simulink model "motorCooling"  (R2025b)
settings: Solver=VariableStepAuto  StartTime=0.0  StopTime=80  RelTol=1e-3  AbsTol=1e-3
PreLoadFcn:
  | load fsDCycle.mat
  | vehicleData
undefined symbols (not defined in the file): battery, bevGear, bevMotorSpdRef, cooling, FL, FR, motorDrive, RL, RR, vehicle
libraries: fl_lib x47, nesl_utility x24, sdl_lib x11, SimscapeFluids_lib x3, ee_lib x2, simulink x1, slpidlib x1, autolibshared x1, batteryecm_lib x1, BatteryEstimators x1
(part 1 of 3)
CloseFcn:
  | try,close(h1_ssc_bev_01),end
  | clear h1_ssc_bev_01
  | try,close(h2_ssc_bev_01),end
  | clear h2_ssc_bev_01
  | try,close(h3_ssc_bev_01),end
  | clear h3_ssc_bev_01
  | try,close(h4_ssc_bev_01),end
  | clear h4_ssc_bev_01
  | 
  | 
  | clear simlog_ssc_bev_01
  | clear logsout_ssc_bev_01
Description:
  | Battery Electric Vehicle, Basic Vehicle
settings Model: Creator=smiller  LastModifiedBy=muizz
settings SolverCC: AutoScaleAbsTol=off  MaxConsecutiveMinStep=2  AlgebraicLoopSolver=TrustRegion
settings DataIOCC: MaxDataPoints=10000  ReturnWorkspaceOutputs=off  SignalLoggingName=logsout_motorCooling
settings OptimizationCC: ReuseModelBlockBuffer=off
settings DebuggingCC: UnconnectedInputMsg=warning  UnconnectedOutputMsg=warning  UnconnectedLineMsg=warning  SymbolicDimsDataTypeCodeGenerationDiagnostic=none
settings ModelReferenceCC: EnableRefExpFcnMdlSchedulingChecks=on
settings SFSimCC: CustomCodeUndefinedFunction=UseInterfaceOnly
settings RTWCC: GPUComputeCapability=3.5  DLArmComputeVersion=19.05
settings SimscapeCC: SimscapeLogType=all  SimscapeLogSimulationStatistics=on  SimscapeLogName=simlog_motorCooling  SimscapeLogDataHistory=300000.0

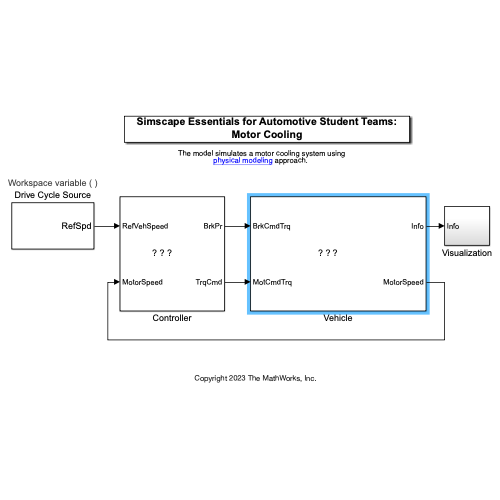
[thumbnail: Simulink's stored preview of the top-level diagram]
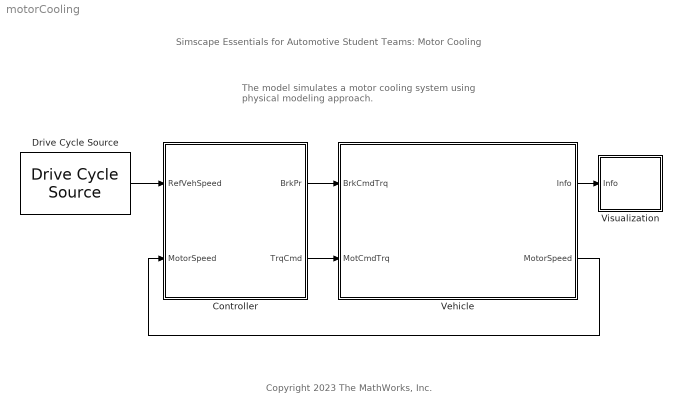
== system motorCooling ==
  note: The model simulates a motor cooling system using physical modeling approach.
  note: Simscape Essentials for Automotive Student Teams: Motor Cooling
  note: Copyright 2023 The MathWorks, Inc.
  Controller : Subsystem
      mask Display: image('Images/brakeThrottle.png'); % Use "Edit Image" on toolstrip to change.
  Drive Cycle Source : autolibshared/Drive Cycle Source  cycleVar=Workspace variable  wsVar=fsdCycle  fileVar=cycleFTP75.mat  tfinal=""  cycleRepeat=on  outAccPort=off  outGearPort=off  gearList=No gear data  t_wot1=5  xdot_woto=0  xdot_wot1=30  t_wot2=20  xdot_wot2=0  t_wotend=30  srcUnit=m/s  outUnit=km/h  srcAccUnit=m/s/s  outAccUnit=m/s^2  dt=0  aMode=1  faultOption=off  velBnd=2  velBndUnit=mph  inUnit=m/s  timeBnd=1  failOption=off  stopSim=off  maxFaultCnt=10  maxFaultTime=2  maxTotFaultTime=15  traceOption=off  dtTrace=1  traceWindow=10  lastDCname=Custom Data Set  lastOutUnit=mph  lastDT=0  lastTB=1  lastSB=2  forceCalcBound=off
  Vehicle : Subsystem
      mask Display: image('Images/vehicle.jpg'); % Use "Edit Image" on toolstrip to change.
  Visualization : Subsystem
  wires:
  Vehicle/2(MotorSpeed) -> Controller/2(MotorSpeed)
  Drive Cycle Source/1 -> Controller/1(RefVehSpeed)
  Vehicle/1(Info) -> Visualization/1(Info)
  Controller/1(BrkPr) -> Vehicle/1(BrkCmdTrq)
  Controller/2(TrqCmd) -> Vehicle/2(MotCmdTrq)

== system motorCooling/Controller ==
  RefVehSpeed : Inport
  MotorSpeed : Inport  Port=2
  Control : Subsystem
      settings: PortSchema="{\"entries\":[{\"content\":{\"sides\":[{\"content\":{\"connectorIds\":[\"Out1\",\"Out2\"]},\"type\":\"ConnectorPlacement.EquallySpacedRectSide\",\"uuid\":\"12b9f2c9-2b28-451b-ad36-7fe4150db485\"},{\"content\":{\"connectorIds\":[\"In1\",\"In2\"],\"side\":\"RIGHT\"},\"type\":\"ConnectorPlacement.EquallySpacedRectSide\",\"uuid\":\"c0fdf9a4-483a-4ddc-b663-6299fcc79327\"},{\"content\":{\"connectorIds\":[],\"side\":\"TOP\"},\"type\":\"ConnectorPlacement.EquallySpacedRectSide\",\"uuid\":\"3f20082e-8487-45e3-9fd7-d6d75741df4d\"}]},\"type\":\"ConnectorPlacement.EquallySpacedConnector\",\"uuid\":\"9361cdd3-74d8-46ee-ae7f-e2dde5d31ed1\"}],\"packageUris\":[\"http://schema.mathworks.com/mf0/Connector/R2020b\"],\"version\":\"1.0\"}"
  Motor Speed Reference : Subsystem
  BrkPr : Outport
  TrqCmd : Outport  Port=2
  tag scope: Ref=global
  wires:
  MotorSpeed/1 -> Control/1(Spd)
  Motor Speed Reference/1(MotorSpdRef) -> Control/2(SpdRef)
  RefVehSpeed/1 -> [Ref], Motor Speed Reference/1(VehSpd)
  Control/1(BrkPr) -> BrkPr/1  "BrkPr"
  Control/2(TrqCmd) -> TrqCmd/1  "MotCmdTrq"

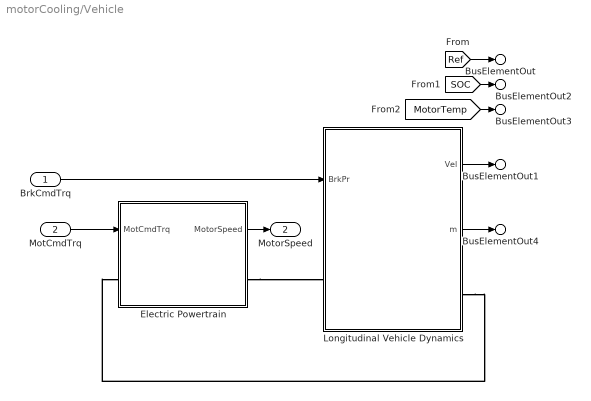
== system motorCooling/Vehicle ==
  BrkCmdTrq : Inport
  MotCmdTrq : Inport  Port=2
  Electric Powertrain : Subsystem
  Longitudinal Vehicle Dynamics : Subsystem
  BusElementOut1 : Outport  PortName=Info  Element=VehSpeed
  BusElementOut : Outport  PortName=Info  Element=RefVehSpeed
  BusElementOut2 : Outport  PortName=Info  Element=SOC
  BusElementOut3 : Outport  PortName=Info  Element=MotorTemp
  BusElementOut4 : Outport  PortName=Info  Element=Vehicle
  MotorSpeed : Outport  Port=2  VectorParamsAs1DForOutWhenUnconnected=off
  wires:
  [Ref] -> BusElementOut/1
  [SOC] -> BusElementOut2/1
  [MotorTemp] -> BusElementOut3/1
  Electric Powertrain/1(MotorSpeed) -> MotorSpeed/1
  BrkCmdTrq/1 -> Longitudinal Vehicle Dynamics/1(BrkPr)
  Longitudinal Vehicle Dynamics/1(Vel) -> BusElementOut1/1
  Longitudinal Vehicle Dynamics/2(m) -> BusElementOut4/1
  MotCmdTrq/1 -> Electric Powertrain/1(MotCmdTrq)
  connections:
  Electric Powertrain/RConn1 -- Longitudinal Vehicle Dynamics/LConn1
  Longitudinal Vehicle Dynamics/RConn1 -- Electric Powertrain/LConn1

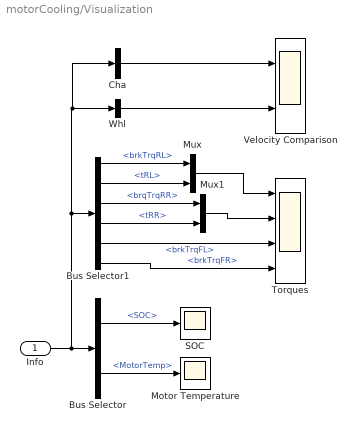
== system motorCooling/Visualization ==
  Info : Inport
  Bus Selector : BusSelector  OutputSignals=SOC,MotorTemp
  Bus Selector1 : BusSelector  OutputSignals=Vehicle.Brakes.RL.brkTrqRL,Vehicle.Chassis.tRL,Vehicle.Brakes.RR.brqTrqRR,Vehicle.Chassis.tRR,Vehicle.Brakes.FL.brkTrqFL,Vehicle.Brakes.FR.brkTrqFR
  Cha : BusSelector  OutputSignals=VehSpeed,RefVehSpeed  OutputAsBus=on
  Motor Temperature : Scope
      settings: ActiveDisplayYMinimum=273.34327  ActiveDisplayYMaximum=321.4106  DataLoggingVariableName=ScopeData3
  Mux : Mux  Inputs=2
  Mux1 : Mux  Inputs=2
  SOC : Scope
      settings: ActiveDisplayYMinimum=0.87315  ActiveDisplayYMaximum=0.90298  DataLoggingVariableName=ScopeData2
  Torques : Scope  NumInputPorts=4
      settings: Title=Rear Left, Brake and Drive Torque  ActiveDisplayYMinimum=-700  ActiveDisplayYMaximum=500
  Velocity Comparison : Scope  NumInputPorts=2
      settings: Title=Vehicle Speed  ActiveDisplayYMinimum=-11.92946  ActiveDisplayYMaximum=107.36516  DataLoggingVariableName=ScopeData2
  Whl : BusSelector  OutputSignals=Vehicle.Brakes.FL.wFL,Vehicle.Brakes.RR.wRR,Vehicle.Brakes.RL.wRL,Vehicle.Brakes.FR.wFR  OutputAsBus=on
  wires:
  Bus Selector/2 -> Motor Temperature/1  "<MotorTemp>"
  Bus Selector/1 -> SOC/1  "<SOC>"
  Whl/1 -> Velocity Comparison/2
  Cha/1 -> Velocity Comparison/1
  Mux1/1 -> Torques/2
  Mux/1 -> Torques/1
  Bus Selector1/4 -> Mux1/2  "<tRR>"
  Bus Selector1/2 -> Mux/2  "<tRL>"
  Bus Selector1/3 -> Mux1/1  "<brqTrqRR>"
  Bus Selector1/1 -> Mux/1  "<brkTrqRL>"
  Bus Selector1/6 -> Torques/4  "<brkTrqFR>"
  Bus Selector1/5 -> Torques/3  "<brkTrqFL>"
  Info/1 -> Cha/1, Whl/1, Bus Selector1/1, Bus Selector/1

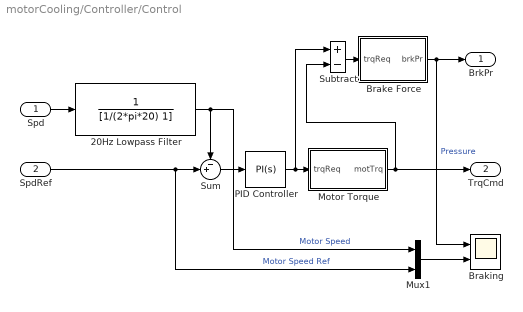
== system motorCooling/Controller/Control ==
  Spd : Inport  Unit=rpm
  SpdRef : Inport  Port=2  Unit=rpm
  20Hz Lowpass Filter : TransferFcn  Denominator=[1/(2*pi*20) 1]
  Brake Force : Subsystem
  Braking : Scope  NumInputPorts=2
      settings: ActiveDisplayYMinimum=-6.26637814618E+6  ActiveDisplayYMaximum=5.639740331562E+7
  Motor Torque : Subsystem
  Mux1 : Mux  Inputs=2
  PID Controller : slpidlib/PID Controller  Controller=PI  Form=Parallel  TimeDomain=Continuous-time  UseExternalTs=off  SampleTime=-1  IntegratorMethod=Forward Euler  FilterMethod=Forward Euler  ControllerParametersSource=internal  P=0.5  I=1e-3  UseKiTs=off  D=0  UseExternalDerivativeSource=off  N=100  UseFilter=on  TunerSelectOption=Transfer Function Based (PID Tuner App)  InitialConditionSource=internal  InitialConditionForIntegrator=0  InitialConditionForFilter=0  DifferentiatorICPrevScaledInput=0  ExternalReset=none  TrackingMode=off  Kt=1  LimitOutput=off  SatLimitsSource=internal  UpperSaturationLimit=inf  LowerSaturationLimit=-inf  LinearizeAsGain=on  AntiWindupMode=none  Kb=1  LimitIntegrator=off  UpperIntegratorSaturationLimit=inf  LowerIntegratorSaturationLimit=-inf  POutMin=[]  POutMax=[]  IOutMin=[]  IOutMax=[]  DOutMin=[]  DOutMax=[]  NOutMin=[]  NOutMax=[]  SumOutMin=[]  SumOutMax=[]  SaturationOutMin=[]  SaturationOutMax=[]  PParamMin=[]  PParamMax=[]  IParamMin=[]  IParamMax=[]  DParamMin=[]  DParamMax=[]  NParamMin=[]  NParamMax=[]  KbParamMin=[]  KbParamMax=[]  KtParamMin=[]  KtParamMax=[]  KbOutMin=[]  KbOutMax=[]  KtOutMin=[]  KtOutMax=[]  IntegratorOutMin=[]  IntegratorOutMax=[]  FilterOutMin=[]  FilterOutMax=[]  SumI1OutMin=[]  SumI1OutMax=[]  SumI2OutMin=[]  SumI2OutMax=[]  SumI3OutMin=[]  SumI3OutMax=[]  SumI4OutMin=[]  SumI4OutMax=[]  SumDOutMin=[]  SumDOutMax=[]  DifferentiatorOutMin=[]  DifferentiatorOutMax=[]  FilterDiffOutCoefMin=[]  FilterDiffOutCoefMax=[]  ReciprocalOutMin=[]  ReciprocalOutMax=[]  SumDenOutMin=[]  SumDenOutMax=[]  SumNumOutMin=[]  SumNumOutMax=[]  DivideOutMin=[]  DivideOutMax=[]  UdiffTsProdOutMin=[]  UdiffTsProdOutMax=[]  NTsProdOutMin=[]  NTsProdOutMax=[]  UintegralTsProdOutMin=[]  UintegralTsProdOutMax=[]  UngainTsProdOutMin=[]  UngainTsProdOutMax=[]  ClampingZeroOutDataTypeStr=Inherit: Inherit via back propagation  ClampingZeroOutMin=[]  ClampingZeroOutMax=[]  FilterDenConstantOutDataTypeStr=Inherit: Inherit via back propagation  FilterDenConstantOutMin=[]  FilterDenConstantOutMax=[]  PCopyOutDataTypeStr=Inherit: Inherit via back propagation  PCopyOutMin=[]  PCopyOutMax=[]  NCopyOutDataTypeStr=Inherit: Inherit via back propagation  NCopyOutMin=[]  NCopyOutMax=[]  IntegratorContinuousStateAttributes=''  IntegratorStateMustResolveToSignalObject=off  IntegratorRTWStateStorageClass=Auto  FilterContinuousStateAttributes=''  FilterStateMustResolveToSignalObject=off  FilterRTWStateStorageClass=Auto  ParallelPVariant=InternalParameters  IdealPVariant=Disabled  IVariant=InternalParameters  DVariant=Disabled  IntegratorVariant=Continuous  SatVariant=Disabled  AWVariant=Passthrough  PCopyVariant=Disabled  TRVariant=Disabled  FdbkBlocksVariant=Forward  IdealPFdbkVariant=Disabled  SatFdbkVariant=Disabled  DerivativeFilterVariant=Disabled  NVariant=Disabled  NCopyVariant=Disabled_SignalSpec  FilterICVariant=Disabled  IntegratorICVariant=InternalICs  ExternalResetVariant=Disabled  TRSumVariant=Passthrough  SumFdbkVariant=Disabled  SumVariant=Sum_PI  TsampFilterVariant=InternalTs  TsampNgainVariant=Passthrough  TsampIntegralVariant=Disabled_SignalSpec  ExternalSaturationOutDataTypeStr=Inherit: Same as second input  DerivativeSourceVariant=Disabled  PreIntVariant=InternalPreInt
  Subtract : Sum  Inputs=+-
  Sum : Sum  Inputs=-+|
  BrkPr : Outport
  TrqCmd : Outport  Port=2  Unit=N*m  VectorParamsAs1DForOutWhenUnconnected=off
  wires:
  20Hz Lowpass Filter/1 -> Sum/1, Mux1/1  "Motor Speed"
  Sum/1 -> PID Controller/1
  Spd/1 -> 20Hz Lowpass Filter/1
  SpdRef/1 -> Mux1/2, Sum/2  "Motor Speed Ref"
  Motor Torque/1(motTrq) -> Subtract/2, TrqCmd/1
  Brake Force/1(brkPr) -> BrkPr/1, Braking/1  "Pressure"
  Subtract/1 -> Brake Force/1(trqReq)
  Mux1/1 -> Braking/2
  PID Controller/1 -> Subtract/1, Motor Torque/1(trqReq)

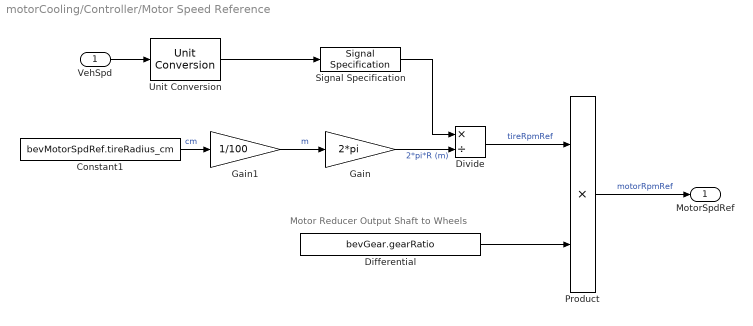
== system motorCooling/Controller/Motor Speed Reference ==
  note: Motor Reducer Output Shaft to Wheels
  VehSpd : Inport  Unit=km/hr
  Constant1 : Constant  Value=bevMotorSpdRef.tireRadius_cm
  Differential : Constant  Value=bevGear.gearRatio
  Divide : Product  Inputs=*/
  Gain : Gain  Gain=2*pi
  Gain1 : Gain  Gain=1/100
  Product : Product
  Signal Specification : SignalSpecification  Unit=m/min
  Unit Conversion : UnitConversion
  MotorSpdRef : Outport  Unit=rpm  VectorParamsAs1DForOutWhenUnconnected=off
  wires:
  VehSpd/1 -> Unit Conversion/1
  Unit Conversion/1 -> Signal Specification/1
  Signal Specification/1 -> Divide/1
  Constant1/1 -> Gain1/1  "cm"
  Gain/1 -> Divide/2  "2*pi*R (m)"
  Divide/1 -> Product/1  "tireRpmRef"
  Product/1 -> MotorSpdRef/1  "motorRpmRef"
  Gain1/1 -> Gain/1  "m"
  Differential/1 -> Product/2

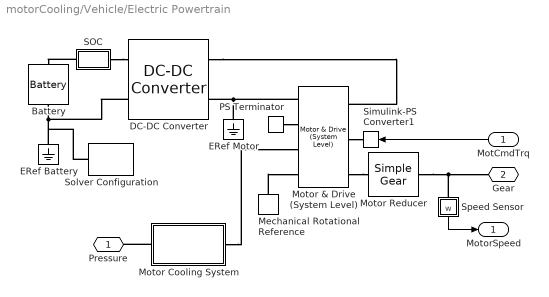
== system motorCooling/Vehicle/Electric Powertrain ==
  MotCmdTrq : Inport
  Battery : batteryecm_lib/Battery  Vnom=battery.voltage_V V  prm_dir=simscape.enum.battery.prm_dir.disabled  R1_dis=2 Ohm  R1_ch=2 Ohm  R1=2e-3 Ohm  prm_AH=simscape.enum.battery.prm_AH.finite  AH=battery.cell_capacity A*hr  V1=battery.voltage_V*11.5/12 V  AH1=10 A*hr  prm_R2=simscape.enum.battery.prm_R2.disabled  R2=2000 Ohm  Tmeas=298.15 K  charge_measurement_port=simscape.enum.battery.enable.no  prm_dyn=simscape.enum.battery.prm_dyn.off  Rp1=0.005 Ohm  tau1=30 s  Rp2=0.005 Ohm  tau2=30 s  Rp3=0.005 Ohm  tau3=30 s  Rp4=0.005 Ohm  tau4=30 s  Rp5=0.005 Ohm  tau5=30 s  prm_fade=simscape.enum.battery.prm_fade.disabled  N_fade=100  AH_fade=45 A*hr  R1_fade=2.02 Ohm  R1_ch_fade=2.02 Ohm  V1_fade=10.35 V  prm_age=simscape.enum.battery.prm_age.disabled  prm_age_OCV=simscape.enum.battery.prm_age_OCV.OCV  OCV_age=0.9  SOC_age=60  Tmeas_age=298.15 K  delta_time_age_vec=[0] d  temperature_age_vec=[273] K  OCV_scaling_age=2.2134e6  OCV_offset_age=1.632e6  temp_exp_age=0.515833569 V  t_exp_age=0.75  Vnom_T2=12 V  R1_T2=2.2 Ohm  R1_T2_dis=2.2 Ohm  R1_T2_ch=2.2 Ohm  V1_T2=11.4 V  R2_T2=2200 Ohm  Rp1_T2=0.005 Ohm  tau1_T2=30 s  Rp2_T2=0.005 Ohm  tau2_T2=30 s  Rp3_T2=0.005 Ohm  tau3_T2=30 s  Rp4_T2=0.005 Ohm  tau4_T2=30 s  Rp5_T2=0.005 Ohm  tau5_T2=30 s  Tmeas2=273.15 K  thermal_port=simscape.enum.thermaleffects.omit  thermal_mass=30000 J/K  i_specify=off  i_priority=None  i=0 A  i_nominal_specify=off  i_nominal_value=1  i_nominal_unit=A  v_specify=off  v_priority=None  v=0 V  v_nominal_specify=off  v_nominal_value=1  v_nominal_unit=V  charge_specify=on  charge_priority=High  charge=battery.cell_capacity*battery.init_soc A*hr  charge_nominal_specify=off  charge_nominal_value=1  charge_nominal_unit=A*hr  num_cycles_specify=off  num_cycles_priority=High  num_cycles=0  num_cycles_nominal_specify=off  num_cycles_nominal_value=1  num_cycles_nominal_unit=1  temperature_specify=off  temperature_priority=High  temperature=298.15 K  temperature_nominal_specify=off  temperature_nominal_value=1  temperature_nominal_unit=K
  DC-DC Converter : ee_lib/Semiconductors & Converters/Converters/DC-DC Converter  Vref_option=ee.enum.converters.voltageref.internal  v_ref=converter.outputVoltage V  P_rated=converter.outputPower W  droop_enabled=true  droop_param=ee.enum.converters.droop.percent  droop=0.1 V/A  droop_percent=converter.droopPercent  Vref_droop=10 V  reversible=ee.enum.converters.directionality.bidirectional  G_diode=1e-8 1/Ohm  P_fixed=1 W  losses_option=ee.enum.converters.lossesOption.proportionalToSquaredCurrent  eff_rated=80  tableOption=ee.enum.converters.lossTableOptionThermal.currentTemp  i_eff_vec=[-2, -1, 1, 2] A  v_eff_vec=[15, 30, 45] V  eff_vec=[66, 76, 80, 74]  eff_2D_table=[66, 66, 66; 76, 76, 76; 80, 80, 80; 74, 74, 74]  model_dynamics=ee.enum.converters.dynamics.no  tau=0.02 s  v_ini=10 V  v1_min=1 V  R1=1000 Ohm  R2=1000 Ohm  fault_condition=ee.enum.faults.faultInputCondition.greaterThan  fault_threshold=0.5  T_eff_vec=[280, 300, 320] K  eff_3D_table=repmat([66; 76; 80; 74], 1, 3, 3)  thermal_mass=100 J/K  initial_temperature=298.15 K
      settings: InternalSimscapePortConfiguration="{\"Bottom\":[],\"Left\":[{\"id\":\"p1\",\"label\":\"1+\",\"type\":\"foundation.electrical.electrical\"},{\"id\":\"n1\",\"label\":\"1-\",\"type\":\"foundation.electrical.electrical\"}],\"Right\":[{\"id\":\"p2\",\"label\":\"2+\",\"type\":\"foundation.electrical.electrical\"},{\"id\":\"n2\",\"label\":\"2-\",\"type\":\"foundation.electrical.electrical\"}],\"Top\":[]}"
  ERef Battery : fl_lib/Electrical/Electrical Elements/Electrical Reference
  ERef Motor : fl_lib/Electrical/Electrical Elements/Electrical Reference
  Mechanical Rotational Reference : fl_lib/Mechanical/Rotational Elements/Mechanical Rotational Reference
  Motor Reducer : sdl_lib/Gears/Simple Gear  ratio=motorDrive.gearRatioCompensation  rotation_direction=3-2*(1)  friction_model=sdl.enum.gear_efficiencies_load.off  T_noload=0.1 N*m  T_nom=5 N*m  efficiency_nom=0.8  efficiency=0.8  temperature_TLU=[280, 300, 320] K  load_TLU=[1, 5, 10] N*m  efficiency_TLU=[.95, .9, .85]  efficiency_TLU2=[.85, .8, .75; .95, .9, .85; .85, .8, .7]  w_thr=0.01 rad/s  pwr_thr=0.001 W  enable_backlash=false  hardstop_model=simscape.enum.hardstop.smooth  backlash_distance=1e-3 mm  r_base=0.1 m  transition=1e-4 mm  backlash_stiffness=1e7 N/m  backlash_damping=1e6 N*s/m  coeff_rest=0  v_tol=0.001 m/s  f_tol=0 N  mu_visc=[0, 0] N*m/(rad/s)  thermal_mass=50 J/K  temperature_specify=off  temperature_priority=High  temperature=300 K  temperature_nominal_specify=off  temperature_nominal_value=1  temperature_nominal_unit=K  x_backlash_specify=off  x_backlash_priority=None  x_backlash=0 mm  x_backlash_nominal_specify=off  x_backlash_nominal_value=1  x_backlash_nominal_unit=mm  f_hardstop_specify=off  f_hardstop_priority=None  f_hardstop=0 N  f_hardstop_nominal_specify=off  f_hardstop_nominal_value=1  f_hardstop_nominal_unit=N  v_backlash_specify=off  v_backlash_priority=None  v_backlash=0 m/s  v_backlash_nominal_specify=off  v_backlash_nominal_value=1  v_backlash_nominal_unit=m/s
  Motor & Drive (System Level) : ee_lib/Electromechanical/Motor & Drive (System Level)  torque_speed_param=ee.enum.electromech.envelope.torque_power  overtorque_param=ee.enum.electromech.overtorque.no  T_t=[.09, .08, .07, 0] N*m  T_t_intermittent=[.36, .32, .28, 0] N*m  T_t_2D=[.09, .09, .09; .08, .08, .08; .07, .07, .07; 0, 0, 0] N*m  T_t_intermittent_2D=[.36, .36, .36; .32, .32, .32; .28, .28, .28; 0, 0, 0] N*m  w_t=[0, 3750, 7500, 8000] rpm  vdc_t=[6, 12, 24] V  torque_max=motorDrive.simplePmsmDrv_trqMax_Nm N*m  power_max=motorDrive.simplePmsmDrv_powMax_W W  torque_max_intermittent=0.4 N*m  power_max_intermittent=120 W  time_overtorque=30 s  time_recover=60 s  Tc=motorDrive.simplePmsmDrv_timeConst_s s  EnableSwitch=simscape.enum.onoff.off  losses_param=2  eff=100  w_eff=3750 rpm  T_eff=0.08 N*m  Piron=0 W  Pbase=0 W  w_eff_vec=motorDrive.simplePmsmDrv_spdVec_rpm rpm  T_eff_vec=motorDrive.simplePmsmDrv_trqVec_Nm N*m  v_eff_vec=[100, 250, 400] V  losses_mat=motorDrive.simplePmsmDrv_LossTbl_W W  efficiency_mat=[95, 95, 95, 95; 95, 95, 95, 95; 95, 95, 95, 95; 95, 95, 95, 95; 95, 95, 95, 95]  losses_mat_3D=ones(5, 4, 3) W  efficiency_mat_3D=95 * ones(5, 4, 3)  Res=0 Ohm  J=motorDrive.simplePmsmDrv_rotorInertia_kg_m2 kg*m^2  lam=motorDrive.simplePmsmDrv_rotorDamping_Nm_per_radps N*m/(rad/s)  speed0=motorDrive.simplePmsmDrv_initialRotorSpd_rpm rpm  faulted_specify=off  faulted_priority=None  faulted=0  faulted_nominal_specify=off  faulted_nominal_value=1  faulted_nominal_unit=1  isSwitchedOff_specify=off  isSwitchedOff_priority=None  isSwitchedOff=0  isSwitchedOff_nominal_specify=off  isSwitchedOff_nominal_value=1  isSwitchedOff_nominal_unit=1  torqueLimitContinuous_specify=off  torqueLimitContinuous_priority=None  torqueLimitContinuous=0 N*m  torqueLimitContinuous_nominal_specify=off  torqueLimitContinuous_nominal_value=1  torqueLimitContinuous_nominal_unit=N*m  alpha=3.93e-3 1/K  Tmeas=25 degC  Tmeas2=125 degC  losses_mat_T2=motorDrive.simplePmsmDrv_LossTbl_W W  efficiency_mat_T2=[95, 95, 95, 95; 95, 95, 95, 95; 95, 95, 95, 95; 95, 95, 95, 95; 95, 95, 95, 95]  losses_mat_3D_T2=ones(5, 4, 3) W  efficiency_mat_3D_T2=95 * ones(5, 4, 3)  thermal_mass=10 J/K  initial_temperature=5 degC
      settings: LogSimulationData=on  InternalSimscapePortConfiguration="{\"Bottom\":[],\"Left\":[{\"id\":\"Vp\",\"label\":\"+\",\"type\":\"foundation.electrical.electrical\"},{\"id\":\"Tr\",\"label\":\"Tr\",\"type\":\"input\"},{\"id\":\"R\",\"label\":\"R\",\"type\":\"foundation.mechanical.rotational.rotational\"}],\"Right\":[{\"id\":\"Vm\",\"label\":\"-\",\"type\":\"foundation.electrical.electrical\"},{\"id\":\"Omega\",\"label\":\"w\",\"type\":\"output\"},{\"id\":\"H\",\"label\":\"H\",\"type\":\"foundation.thermal.thermal\"},{\"id\":\"C\",\"label\":\"C\",\"type\":\"foundation.mechanical.rotational.rotational\"}],\"Top\":[]}"
  Motor Cooling System : Subsystem
  PS Terminator : fl_lib/Physical Signals/Sinks/PS Terminator
  SOC : Subsystem
  Simulink-PS Converter1 : nesl_utility/Simulink-PS Converter  PhysicalDomain=network_engine_domain  SubClassName=ps_input  LeftPortType=input  RightPortType=output  PseudoPeriodic=off  Frequencies=[]  NoiseDistribution=none  NoiseParameters=[]  Unit=N*m  AffineConversion=off  FilteringAndDerivatives=provide  SimscapeFilterOrder=1  InputFilterTimeConstant=0.001  UdotUserProvided=0
  Solver Configuration : nesl_utility/Solver Configuration  PhysicalDomain=network_engine_domain  SubClassName=solver  LeftPortType=input  RightPortType=generic  Tones=[]  Harmonics=[]  SimulateNoise=off  Profile=off  UseLocalSampling=off  EnableSwitchedLinearOptims=on  FrequencyDomain=off  UseCCode=off  RelTol=0.001  AbsTol=1e-06  MinStep=1e-09  ToWorkspace=off  RevertToSquareIcSolve=off  NumHomotopyIterations=100  PhasorMode=off  PhasorModeNumHarmonics=1  ConsistencySolver=NEWTON_FTOL  IndexReductionMethod=DerivativeReplacement  DoDC=off  ResidualTolerance=1e-09  ConsistencyTolSource=GLOBAL  ConsistencyAbsTol=0.001  ConsistencyRelTol=0.001  ConsistencyTolFactor=0.001  UseLocalSolver=off  LocalSolverChoice=NE_BACKWARD_EULER_ADVANCER  ResolveIndetEquations=on  FunctionEvalNumThread=1  LocalSolverSampleTime=0.001  DoFixedCost=off  MaxNonlinIter=3  MaxModeIter=2  ComputeImpulses=off  ImpulseIterations=2  LinearAlgebra=auto  LinearAlgebraNumThread=0  EquationFormulation=NE_TIME_EF  DelaysMemoryBudget=1024  AutomaticFiltering=on  FilteringTimeConstant=0.001  PartitionStorageMethod=AS_NEEDED  PartitionMemoryBudget=1024  PartitionMethod=ROBUST  MultibodyUseLocalSolver=off  MultibodyLocalSolverChoice=ODE1  MultibodyLocalSolverSampleTime=0.001
  Speed Sensor : Subsystem
      mask Display: disp('w')
  Pressure : PMIOPort  Side=Left
  Gear : PMIOPort  Port=2  Side=Right
  MotorSpeed : Outport
  wires:
  Speed Sensor/1(w) -> MotorSpeed/1
  MotCmdTrq/1 -> Simulink-PS Converter1/1
  connections:
  Motor & Drive (System Level)/RConn1 -- ERef Motor/LConn1 -- DC-DC Converter/RConn2
  DC-DC Converter/RConn1 -- Motor & Drive (System Level)/LConn1
  Motor & Drive (System Level)/LConn2 -- Simulink-PS Converter1/RConn1
  Mechanical Rotational Reference/LConn1 -- Motor & Drive (System Level)/RConn4
  SOC/RConn1 -- DC-DC Converter/LConn1
  Motor Cooling System/LConn1 -- Motor & Drive (System Level)/RConn3
  Motor & Drive (System Level)/LConn3 -- Motor Reducer/LConn1
  Motor Cooling System/RConn1 -- Pressure/RConn1
  PS Terminator/LConn1 -- Motor & Drive (System Level)/RConn2
  Motor Reducer/RConn1 -- Gear/RConn1 -- Speed Sensor/LConn1
  SOC/LConn1 -- Battery/LConn1
  DC-DC Converter/LConn2 -- Solver Configuration/RConn1 -- ERef Battery/LConn1 -- Battery/RConn1

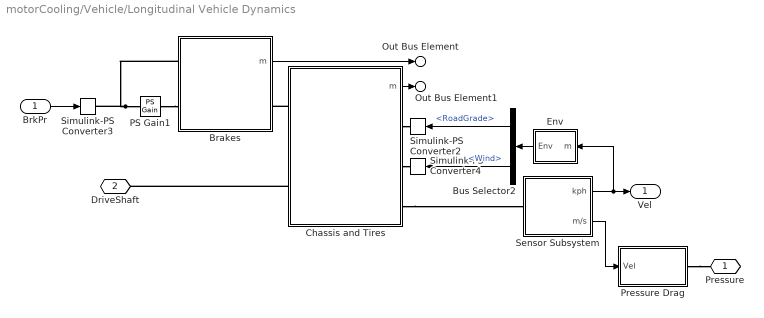
== system motorCooling/Vehicle/Longitudinal Vehicle Dynamics ==
  BrkPr : Inport
  Brakes : Subsystem
  Bus Selector2 : BusSelector  OutputSignals=RoadGrade,Wind
  Chassis and Tires : Subsystem
  Env : Subsystem
  PS Gain1 : fl_lib/Physical Signals/Functions/PS Gain  gain=1
  Pressure Drag : Subsystem
  Sensor Subsystem : Subsystem
  Simulink-PS Converter2 : nesl_utility/Simulink-PS Converter  PhysicalDomain=network_engine_domain  SubClassName=ps_input  LeftPortType=input  RightPortType=output  PseudoPeriodic=off  Frequencies=[]  NoiseDistribution=none  NoiseParameters=[]  Unit=rad  AffineConversion=off  FilteringAndDerivatives=provide  SimscapeFilterOrder=1  InputFilterTimeConstant=0.001  UdotUserProvided=0
  Simulink-PS Converter3 : nesl_utility/Simulink-PS Converter  PhysicalDomain=network_engine_domain  SubClassName=ps_input  LeftPortType=input  RightPortType=output  PseudoPeriodic=off  Frequencies=[]  NoiseDistribution=none  NoiseParameters=[]  Unit=N/m^2  AffineConversion=off  FilteringAndDerivatives=provide  SimscapeFilterOrder=1  InputFilterTimeConstant=0.001  UdotUserProvided=0
  Simulink-PS Converter4 : nesl_utility/Simulink-PS Converter  PhysicalDomain=network_engine_domain  SubClassName=ps_input  LeftPortType=input  RightPortType=output  PseudoPeriodic=off  Frequencies=[]  NoiseDistribution=none  NoiseParameters=[]  Unit=m/s  AffineConversion=off  FilteringAndDerivatives=provide  SimscapeFilterOrder=1  InputFilterTimeConstant=0.001  UdotUserProvided=0
  Pressure : PMIOPort  Side=Right
  DriveShaft : PMIOPort  Port=2  Side=Left
  Vel : Outport
  Out Bus Element : Outport  Port=2  PortName=m  Element=Brakes
  Out Bus Element1 : Outport  Port=2  PortName=m  Element=Chassis
  wires:
  BrkPr/1 -> Simulink-PS Converter3/1
  Env/1(Env) -> Bus Selector2/1
  Brakes/1(m) -> Out Bus Element/1
  Bus Selector2/2 -> Simulink-PS Converter4/1  "<Wind>"
  Bus Selector2/1 -> Simulink-PS Converter2/1  "<RoadGrade>"
  Chassis and Tires/1(m) -> Out Bus Element1/1
  Sensor Subsystem/2(m/s) -> Pressure Drag/1(Vel)
  Sensor Subsystem/1(kph) -> Vel/1, Env/1(m)
  connections:
  Pressure Drag/RConn1 -- Pressure/RConn1
  PS Gain1/LConn1 -- Brakes/LConn1 -- Simulink-PS Converter3/RConn1
  Chassis and Tires/RConn2 -- Simulink-PS Converter4/RConn1
  PS Gain1/RConn1 -- Brakes/LConn2
  Chassis and Tires/LConn2 -- DriveShaft/RConn1
  Chassis and Tires/LConn1 -- Brakes/RConn1
  Chassis and Tires/RConn1 -- Simulink-PS Converter2/RConn1
  Chassis and Tires/RConn3 -- Sensor Subsystem/LConn1

== system motorCooling/Controller/Control/Brake Force ==
  note: Convert requested braking torque to brake pressure
  trqReq : Inport
  Only Negative Trq : Saturate  UpperLimit=0  LowerLimit=-inf  ZeroCross=off
  trq2pressure : Gain  Gain=-3.3e6
  brkPr : Outport
  wires:
  Only Negative Trq/1 -> trq2pressure/1
  trq2pressure/1 -> brkPr/1
  trqReq/1 -> Only Negative Trq/1  "trqReq"

== system motorCooling/Controller/Control/Motor Torque ==
  note: Full torque for acceleration,
      | limited torque for deceleration (regenerative torque)
  trqReq : Inport
  Compare To Zero : simulink/Logic and Bit Operations/Compare To Zero  relop=>  OutDataTypeStr=boolean  ZeroCross=off
  Gain accel torque : Constant
  Gain decel torque : Constant  Value=0.3
  Product : Product
  Saturation Motor Torque Limits : Saturate  UpperLimit=motorDrive.simplePmsmDrv_trqMax_Nm  LowerLimit=motorDrive.simplePmsmDrv_trqMin_Nm
  Switch : Switch  Criteria=u2 > Threshold  SaturateOnIntegerOverflow=off  InputSameDT=off
  motTrq : Outport
  wires:
  Gain decel torque/1 -> Switch/3
  Switch/1 -> Product/1
  Gain accel torque/1 -> Switch/1
  Compare To Zero/1 -> Switch/2
  trqReq/1 -> Product/2, Compare To Zero/1
  Product/1 -> Saturation Motor Torque Limits/1
  Saturation Motor Torque Limits/1 -> motTrq/1
